simulink model "Electrical_System_2018b_obfs"  (R2019b)
settings: Solver=VariableStepAuto  StartTime=0.0  StopTime=5  RelTol=1e-3  AbsTol=1e-3  EnableMultiTasking=on
InitFcn:
  | Steady_State_Initialisation;
StopFcn:
  | %sscexplore(simlog);
  | %Logging
undefined symbols (not defined in the file): abrlhklxvp, aexgmhuedq, afmfmjnutg, afpphrjpnc, ahuxbyvruc, alarvljztt, amxnyqmnuw, aodrlwvqie, aolhmuplyq, aqpmguuqkg, auesgwirzl, aurophlnng, awamelrhru, ayfhvxflxn, azxkacuhqc, babszerikg, bawhdqanwq, bevoqecvei, bltjvqbchx, bmqsuewujl, bsmyqjfgnf, btvjbsmnve, bywgxqeadw, bziaduxaer, bzmcmdqocb, bzsvyvetat, ccsjnrbsih, cdvenygxwh, cedkrnslhx, cjheorclzs, cjrdshrtqx, ckhavyhcza, ckxewznhlz, cmrcgyiplk, conenicnws, cqkejbgjnn, csfnuwymhe, cunupkhwbh, cwzfvzuxxh, dcadmadufn, dcfponivnv, ddtrqjrhjn, dfhoxvkqas, dfrhtcwpne, dfvomcagjv, djijwylxea, dnmeqksrrm, dnzewbdkaa, dsqcykyxav, dtswwlttmm, ecumpidjtv, edegaywrct, ejjjsmnejc, eknqnehjdz, emvdetzouf, esxbqkbahr, etnkkbreiq, eunoiiiirw, ewewcuedir, fatkfxdhtc ... (+386)
libraries: fl_lib x802, ee_lib x362, fl_ps_legacy_lib x160, nesl_utility x85
(part 23 of 26)

== system Electrical_System_2018b_obfs/Redacted_1221/Redacted_7996/Redacted_9242/Redacted_38/Redacted_8107/Redacted_6003 ==
  Redacted_1930 : ee_lib/Passive/Thermal/Thermal Resistor  R=hnrivnapaq K/W  T_specify=off  T_priority=None  T=fdmzqhuwsh K  T_nominal_specify=off  T_nominal_unit=K  T_nominal_value=tdgakkaysy  Q_specify=off  Q_priority=None  Q=cbfpwknynd W  Q_nominal_specify=off  Q_nominal_unit=W  Q_nominal_value=hqcrpimszr
      settings: SourceProductName=Simscape Electrical  SourceProductBaseCode=PS  InternalSimscapePortConfiguration="{\"Bottom\":[],\"Left\":[{\"id\":\"A\",\"label\":\"A\",\"type\":\"foundation.thermal.thermal\"}],\"Right\":[{\"id\":\"B\",\"label\":\"B\",\"type\":\"foundation.thermal.thermal\"}],\"Top\":[]}"
  Redacted_2034 : ee_lib/Semiconductors & Converters/Diode  ModelType=qljxbksejb  Vf=iqtxyhzmad V  Ron=mjyptxjlpj Ohm  Goff=eaiuifgbtc S  prmExp=uovsjyapqx  I12=dfdowkcjum A  V12=mowyumyzjz V  IS=paoryjpoxj A  ec=cwojkwmiiz  I1=oyldfbivbv A  V1=dvertrfmvh V  RS=oebupxhqwy Ohm  Tmeas=latpbskjvi degC  N_series=jdrtgiwiug  N_parallel=kjrtfcnnzv  Rz=ecpdxtdyqu Ohm  BV=regbijmtbt V  C_param=crvhucdqdf  CJ=qdbprudfuu pF  CJ0=zczssgvpsu pF  VJ=fxytmivhee V  Mgrad=hqduwwifxd  Vvec=oeuqtgaaxn V  Cvec=gpqahbkocz pF  FC=siouyjskbk  Q_param=mdplkdbvxr  iRM=iffbbljxua A  iF=pfyoxsblfu A  didt=amrzuaxosg A/us  trr_factor=mnaixlwtuy  trr=zhpnzyhtrk ns  Qrr=zinteenzdg s*uA  TT=leubpgkgse ns  tau=mvtjoetwfm ns  T_param=beccsadefd  IS_T2=gikgczwyer A  I1_T2=ejowqnzasa A  V1_T2=boqexodrvc V  Tmeas2=sekozcasvt degC  EG_param=zvetvjcbns  EG=yfbumhzpta eV  XTI_param=kndiutgvbc  XTI=dmkgiicoqh  dBVdT=sjrqiebaep V/K  Tdevice=zbzjxdappo degC  i_specify=off  i_priority=None  i=pkgkjaaiux A  i_nominal_specify=off  i_nominal_unit=A  i_nominal_value=iqyazggtza  v_specify=off  v_priority=None  v=aqbrsijarw V  v_nominal_specify=off  v_nominal_unit=V  v_nominal_value=rbvnzvqoqw  i_capacitor_specify=off  i_capacitor_priority=None  i_capacitor=tuynidlyyy A  i_capacitor_nominal_specify=off  i_capacitor_nominal_unit=A  i_capacitor_nominal_value=vgeutllmom  v_capacitor_specify=off  v_capacitor_priority=None  v_capacitor=aumsjdybje V  v_capacitor_nominal_specify=off  v_capacitor_nominal_unit=V  v_capacitor_nominal_value=ylnkaqxxjx  power_dissipated_specify=off  power_dissipated_priority=None  power_dissipated=bkghkxdvlu W  power_dissipated_nominal_specify=off  power_dissipated_nominal_unit=W  power_dissipated_nominal_value=zgsnnsunjp  thermal_network_parameterization=nlxrhefnye  Rth=wenpkeadfs K/W  Rth_Foster=pmnajvgqrg K/W  thermal_mass_parameterization=bvpebdmwnx  thermal_mass=tsjtvgxgqo J/K  thermal_mass_Foster=juyxynizkb J/K  thermal_time_constant=tldqxfdatu s  thermal_time_constant_Foster=jovrtdhtnc s  thermal_mass_initial_temperatures=ikqngtdwsm degC
      settings: SourceProductName=Simscape Electrical  InternalSimscapePortConfiguration="{\"Bottom\":[],\"Left\":[{\"id\":\"p\",\"label\":\"\",\"type\":\"foundation.electrical.electrical\"},{\"id\":\"H\",\"label\":\"H\",\"type\":\"foundation.thermal.thermal\"}],\"Right\":[{\"id\":\"n\",\"label\":\"\",\"type\":\"foundation.electrical.electrical\"}],\"Top\":[]}"
  Redacted_2189 : fl_lib/Electrical/Electrical Elements/Switch  R_closed=foccbyagpm Ohm  G_open=qmhdlwyqas 1/Ohm  Threshold=mzryhutpxu  i_specify=off  i_priority=None  i=ronjclvfae A  i_nominal_specify=off  i_nominal_unit=A  i_nominal_value=pepihfswvq  v_specify=off  v_priority=None  v=riglalheal V  v_nominal_specify=off  v_nominal_unit=V  v_nominal_value=llodcbplhq
      settings: SourceProductName=Simscape
  Redacted_2683 : ee_lib/Semiconductors & Converters/Diode  ModelType=unqcuhngcz  Vf=ptgyrbybxg V  Ron=tponyfjprp Ohm  Goff=glxtjcdqxv S  prmExp=cjjxbqorob  I12=tmuirimiso A  V12=ajfpvmmvif V  IS=npqaesggkw A  ec=xhdbjedinc  I1=bhqghsexhn A  V1=kekbinqgmi V  RS=vctdzuibfy Ohm  Tmeas=ywtwqwngjn degC  N_series=ugxhiounyu  N_parallel=txdvgcjciy  Rz=prvnlkeyws Ohm  BV=wsyzieqjme V  C_param=dtqzgbyoxb  CJ=bhponiftbz pF  CJ0=lvxihytxjc pF  VJ=kcfldgdrdj V  Mgrad=ogjcpcefgy  Vvec=sngqltjsza V  Cvec=dibfbaeuxm pF  FC=qlgqcocgqi  Q_param=yhsbhadtka  iRM=vjjdgkalgm A  iF=shtzyfzyvn A  didt=hzdjajnwwy A/us  trr_factor=kikgszlwgz  trr=qxsglffrkr ns  Qrr=dtdzjmwoid s*uA  TT=hvrjrtimqi ns  tau=wsjufvhwdd ns  T_param=ieyyqxgorr  IS_T2=mxbsaftenk A  I1_T2=tkyvlqhfkw A  V1_T2=jubvikjjyh V  Tmeas2=kgfbpqicfn degC  EG_param=gliqfynxcq  EG=jzcujindyz eV  XTI_param=xhknqrejda  XTI=jxihwgswbm  dBVdT=ubhxpvgdyz V/K  Tdevice=hhsxnkxagz degC  i_specify=off  i_priority=None  i=igpuapigbx A  i_nominal_specify=off  i_nominal_unit=A  i_nominal_value=nodxoezgzy  v_specify=off  v_priority=None  v=nkzepssinp V  v_nominal_specify=off  v_nominal_unit=V  v_nominal_value=zdhnmmkhdr  i_capacitor_specify=off  i_capacitor_priority=None  i_capacitor=jiuqpxnscm A  i_capacitor_nominal_specify=off  i_capacitor_nominal_unit=A  i_capacitor_nominal_value=fsbzkpldhi  v_capacitor_specify=off  v_capacitor_priority=None  v_capacitor=wrspuopelq V  v_capacitor_nominal_specify=off  v_capacitor_nominal_unit=V  v_capacitor_nominal_value=wizxjlevyq  power_dissipated_specify=off  power_dissipated_priority=None  power_dissipated=moohbwshzg W  power_dissipated_nominal_specify=off  power_dissipated_nominal_unit=W  power_dissipated_nominal_value=orjgoavjlp  thermal_network_parameterization=vpzbbzxpak  Rth=pqattronql K/W  Rth_Foster=xvgcrkjmlg K/W  thermal_mass_parameterization=jjcteiernu  thermal_mass=nxbznqnvge J/K  thermal_mass_Foster=ykxufvckjj J/K  thermal_time_constant=jhthmobbgu s  thermal_time_constant_Foster=fxwuqslxsp s  thermal_mass_initial_temperatures=ciwlrmaqcf degC
      settings: SourceProductName=Simscape Electrical  InternalSimscapePortConfiguration="{\"Bottom\":[],\"Left\":[{\"id\":\"p\",\"label\":\"\",\"type\":\"foundation.electrical.electrical\"},{\"id\":\"H\",\"label\":\"H\",\"type\":\"foundation.thermal.thermal\"}],\"Right\":[{\"id\":\"n\",\"label\":\"\",\"type\":\"foundation.electrical.electrical\"}],\"Top\":[]}"
  Redacted_3015 : ee_lib/Passive/Thermal/Thermal Resistor  R=bsmyqjfgnf K/W  T_specify=off  T_priority=None  T=oqpnlzayxz K  T_nominal_specify=off  T_nominal_unit=K  T_nominal_value=iwtobpvuwc  Q_specify=off  Q_priority=None  Q=ktnxgmfrmp W  Q_nominal_specify=off  Q_nominal_unit=W  Q_nominal_value=upzdrzoogn
      settings: SourceProductName=Simscape Electrical  SourceProductBaseCode=PS  InternalSimscapePortConfiguration="{\"Bottom\":[],\"Left\":[{\"id\":\"A\",\"label\":\"A\",\"type\":\"foundation.thermal.thermal\"}],\"Right\":[{\"id\":\"B\",\"label\":\"B\",\"type\":\"foundation.thermal.thermal\"}],\"Top\":[]}"
  Redacted_3979 : ee_lib/Passive/Thermal/Thermal Resistor  R=rvpgyzkerd K/W  T_specify=off  T_priority=None  T=gamyhprnkw K  T_nominal_specify=off  T_nominal_unit=K  T_nominal_value=xdfqlvauja  Q_specify=off  Q_priority=None  Q=pitpazxbtg W  Q_nominal_specify=off  Q_nominal_unit=W  Q_nominal_value=xyddpdwmaj
      settings: SourceProductName=Simscape Electrical  SourceProductBaseCode=PS  InternalSimscapePortConfiguration="{\"Bottom\":[],\"Left\":[{\"id\":\"A\",\"label\":\"A\",\"type\":\"foundation.thermal.thermal\"}],\"Right\":[{\"id\":\"B\",\"label\":\"B\",\"type\":\"foundation.thermal.thermal\"}],\"Top\":[]}"
  Redacted_5139 : ee_lib/Passive/Thermal/Thermal Resistor  R=kgzasefujm K/W  T_specify=off  T_priority=None  T=glpeopccez K  T_nominal_specify=off  T_nominal_unit=K  T_nominal_value=jyjirvlwob  Q_specify=off  Q_priority=None  Q=zftpgcvoga W  Q_nominal_specify=off  Q_nominal_unit=W  Q_nominal_value=zlepoxtjjd
      settings: SourceProductName=Simscape Electrical  SourceProductBaseCode=PS  InternalSimscapePortConfiguration="{\"Bottom\":[],\"Left\":[{\"id\":\"A\",\"label\":\"A\",\"type\":\"foundation.thermal.thermal\"}],\"Right\":[{\"id\":\"B\",\"label\":\"B\",\"type\":\"foundation.thermal.thermal\"}],\"Top\":[]}"
  Redacted_5625 : fl_lib/Electrical/Electrical Elements/Switch  R_closed=hyxbklyhaw Ohm  G_open=ewgpjrxxtl 1/Ohm  Threshold=kbwhlogzhf  i_specify=off  i_priority=None  i=qjupciitbk A  i_nominal_specify=off  i_nominal_unit=A  i_nominal_value=zfpqhtzgkw  v_specify=off  v_priority=None  v=hqlzplneaj V  v_nominal_specify=off  v_nominal_unit=V  v_nominal_value=obbwqmtbii
      settings: SourceProductName=Simscape
  Redacted_5657 : ee_lib/Semiconductors & Converters/Diode  ModelType=bbawzmmnac  Vf=cfeosnswqd V  Ron=xmclnzzcel Ohm  Goff=mrxxabbkuw S  prmExp=mirycngfdn  I12=rqbalgkwyr A  V12=tabgwshiiq V  IS=ngrjfbjvvt A  ec=clnbffkkko  I1=rfqzpiiomz A  V1=xfqgijkqbu V  RS=zkaypxwvif Ohm  Tmeas=itkruelsvv degC  N_series=uufuremtuo  N_parallel=exbmquirgy  Rz=hgacsasgax Ohm  BV=bjsuhtbcxp V  C_param=auhmigqxzs  CJ=cyxjnvuiff pF  CJ0=nbcujpgwhf pF  VJ=zjdaaxugeg V  Mgrad=afzrqsjezb  Vvec=dsmzskpzrd V  Cvec=bliaftztkk pF  FC=esociklonl  Q_param=skjwelkzxv  iRM=tmfsjklyvt A  iF=cpuezbuqmz A  didt=himvddlotl A/us  trr_factor=pxnmftscld  trr=etvqnrzcrj ns  Qrr=wjswiowekh s*uA  TT=ataufdbeyn ns  tau=zrchcgagyg ns  T_param=gchzwopuhg  IS_T2=xckwpzlhlc A  I1_T2=avbcowntxa A  V1_T2=gdqqwmkozg V  Tmeas2=quzccqydmr degC  EG_param=myyrsafqxx  EG=bylhplcusy eV  XTI_param=tgzqrnxeqr  XTI=fgzgpgaqen  dBVdT=ipxpuexfni V/K  Tdevice=vftflwilyl degC  i_specify=off  i_priority=None  i=mawfnjxacl A  i_nominal_specify=off  i_nominal_unit=A  i_nominal_value=piuvggfdrd  v_specify=off  v_priority=None  v=hcyikizcwq V  v_nominal_specify=off  v_nominal_unit=V  v_nominal_value=gijzssrjyy  i_capacitor_specify=off  i_capacitor_priority=None  i_capacitor=pydmjkdgai A  i_capacitor_nominal_specify=off  i_capacitor_nominal_unit=A  i_capacitor_nominal_value=gaywohzkxq  v_capacitor_specify=off  v_capacitor_priority=None  v_capacitor=jfxdvraffy V  v_capacitor_nominal_specify=off  v_capacitor_nominal_unit=V  v_capacitor_nominal_value=vhdgjoecmz  power_dissipated_specify=off  power_dissipated_priority=None  power_dissipated=ygmcgoonkr W  power_dissipated_nominal_specify=off  power_dissipated_nominal_unit=W  power_dissipated_nominal_value=lsosbnwnhl  thermal_network_parameterization=uqxbruktsl  Rth=xaazvoxkzm K/W  Rth_Foster=ypbknnzits K/W  thermal_mass_parameterization=krtbkpmofw  thermal_mass=kqhtsapotn J/K  thermal_mass_Foster=snricxyamm J/K  thermal_time_constant=dsoiduioti s  thermal_time_constant_Foster=hjownphtlb s  thermal_mass_initial_temperatures=cbnczxkoai degC
      settings: SourceProductName=Simscape Electrical  InternalSimscapePortConfiguration="{\"Bottom\":[],\"Left\":[{\"id\":\"p\",\"label\":\"\",\"type\":\"foundation.electrical.electrical\"},{\"id\":\"H\",\"label\":\"H\",\"type\":\"foundation.thermal.thermal\"}],\"Right\":[{\"id\":\"n\",\"label\":\"\",\"type\":\"foundation.electrical.electrical\"}],\"Top\":[]}"
  Redacted_618 : ee_lib/Semiconductors & Converters/Diode  ModelType=rkpcosdcop  Vf=lzenazmxwk V  Ron=laoauccyph Ohm  Goff=eogfajxjvg S  prmExp=auhrcuewvk  I12=ephdqsweto A  V12=ybwxgsrgvn V  IS=ehwksjpkam A  ec=giupratzer  I1=shazrtegll A  V1=demzikmedl V  RS=tvlssdjwwv Ohm  Tmeas=ubohgymfpi degC  N_series=ipthgzwmna  N_parallel=bktxcarwhu  Rz=yhyrdpsjtm Ohm  BV=hfwqlzcjfg V  C_param=hapevfajvk  CJ=xwrwppuobh pF  CJ0=yyhmqjagfv pF  VJ=zdzkwausfz V  Mgrad=qxmsnreivi  Vvec=lfikgaftwv V  Cvec=xuowrvsncr pF  FC=unjvmmuvtr  Q_param=rddstsxnsr  iRM=fdsnqcchmj A  iF=fmpnloxlqx A  didt=kwjfevuvbi A/us  trr_factor=zfgybtwped  trr=xqkhnstkiy ns  Qrr=hybyujvqwm s*uA  TT=rgwrqignxd ns  tau=yyhbogviix ns  T_param=kercwremhv  IS_T2=boophnoohc A  I1_T2=acskstwime A  V1_T2=wnwbyhilui V  Tmeas2=tblacebvdl degC  EG_param=fgmqmmniev  EG=jvgkdvfiqn eV  XTI_param=tozzwxdtkj  XTI=fufkmkxntk  dBVdT=jhryqncwej V/K  Tdevice=vcluzljkyb degC  i_specify=off  i_priority=None  i=vattghsfci A  i_nominal_specify=off  i_nominal_unit=A  i_nominal_value=qbkpgcrxyx  v_specify=off  v_priority=None  v=nhxoerlgyg V  v_nominal_specify=off  v_nominal_unit=V  v_nominal_value=uyxtmtfxck  i_capacitor_specify=off  i_capacitor_priority=None  i_capacitor=yvkpdlpfsk A  i_capacitor_nominal_specify=off  i_capacitor_nominal_unit=A  i_capacitor_nominal_value=vbrriwgque  v_capacitor_specify=off  v_capacitor_priority=None  v_capacitor=rzfflaghjc V  v_capacitor_nominal_specify=off  v_capacitor_nominal_unit=V  v_capacitor_nominal_value=uwtguigmwf  power_dissipated_specify=off  power_dissipated_priority=None  power_dissipated=jrdwwynqio W  power_dissipated_nominal_specify=off  power_dissipated_nominal_unit=W  power_dissipated_nominal_value=wbkqdktlnr  thermal_network_parameterization=jpsdwhgqsa  Rth=brlvhyneff K/W  Rth_Foster=vfuijyzesi K/W  thermal_mass_parameterization=phbeyounnd  thermal_mass=dtprcnswbr J/K  thermal_mass_Foster=medownhbcv J/K  thermal_time_constant=zqahowncoh s  thermal_time_constant_Foster=wjifmgurkv s  thermal_mass_initial_temperatures=wlgtjerxmc degC
      settings: SourceProductName=Simscape Electrical  InternalSimscapePortConfiguration="{\"Bottom\":[],\"Left\":[{\"id\":\"p\",\"label\":\"\",\"type\":\"foundation.electrical.electrical\"},{\"id\":\"H\",\"label\":\"H\",\"type\":\"foundation.thermal.thermal\"}],\"Right\":[{\"id\":\"n\",\"label\":\"\",\"type\":\"foundation.electrical.electrical\"}],\"Top\":[]}"
  Redacted_713 : ee_lib/Semiconductors & Converters/Diode  ModelType=lkkcmgpbdm  Vf=bawajenmku V  Ron=kxerbojczb Ohm  Goff=omaqvwbgjm S  prmExp=mhvrvxvkqj  I12=vvcjszndgf A  V12=gwdnghxxjm V  IS=lwabrrpbjq A  ec=sqrpdlrsmb  I1=lmbkodwwso A  V1=xbfckrfhqq V  RS=expttalfyo Ohm  Tmeas=jijdjutikz degC  N_series=shguxfrayi  N_parallel=bjkplhfybw  Rz=iubaophvns Ohm  BV=yekwptqxqa V  C_param=rpswauztdx  CJ=farklfmilj pF  CJ0=sqgevuhphp pF  VJ=dlwsmbukmv V  Mgrad=dkyayzzgyw  Vvec=tsbwaimylc V  Cvec=mmqbanhdym pF  FC=tjmqolgjus  Q_param=tlwfgmybcc  iRM=dsozwffbqo A  iF=qoboxqhvid A  didt=xsxvbubgdx A/us  trr_factor=hpdsygyelk  trr=nuzrdvgkrj ns  Qrr=bidvofxoqv s*uA  TT=jbqeqqkgiu ns  tau=cdcbpkkbne ns  T_param=dqwwjegyew  IS_T2=nufxlxaznm A  I1_T2=tystfaaiyc A  V1_T2=zneeizlvme V  Tmeas2=qcubydlkcn degC  EG_param=kzeqebsucu  EG=nmfdxrvqqk eV  XTI_param=rdqutjekkf  XTI=yxstlhwzsc  dBVdT=dfsxohafhi V/K  Tdevice=tjtorimxyl degC  i_specify=off  i_priority=None  i=fyyxyedswg A  i_nominal_specify=off  i_nominal_unit=A  i_nominal_value=lvqvmsrgcq  v_specify=off  v_priority=None  v=lfxrhfhldc V  v_nominal_specify=off  v_nominal_unit=V  v_nominal_value=ahxasjhyix  i_capacitor_specify=off  i_capacitor_priority=None  i_capacitor=sxezhempdb A  i_capacitor_nominal_specify=off  i_capacitor_nominal_unit=A  i_capacitor_nominal_value=oleoyenlww  v_capacitor_specify=off  v_capacitor_priority=None  v_capacitor=vkfdkqfqeh V  v_capacitor_nominal_specify=off  v_capacitor_nominal_unit=V  v_capacitor_nominal_value=sppyhpvyds  power_dissipated_specify=off  power_dissipated_priority=None  power_dissipated=qxpynkfasn W  power_dissipated_nominal_specify=off  power_dissipated_nominal_unit=W  power_dissipated_nominal_value=wuwbigxvpe  thermal_network_parameterization=vnxrsoiwal  Rth=xnfauzfygo K/W  Rth_Foster=omfzlihdit K/W  thermal_mass_parameterization=vyjchpsxmq  thermal_mass=jkxmnrnghg J/K  thermal_mass_Foster=voiyfowxdv J/K  thermal_time_constant=sluohzzprg s  thermal_time_constant_Foster=hfrqbgktbf s  thermal_mass_initial_temperatures=oxayzqemir degC
      settings: SourceProductName=Simscape Electrical  InternalSimscapePortConfiguration="{\"Bottom\":[],\"Left\":[{\"id\":\"p\",\"label\":\"\",\"type\":\"foundation.electrical.electrical\"},{\"id\":\"H\",\"label\":\"H\",\"type\":\"foundation.thermal.thermal\"}],\"Right\":[{\"id\":\"n\",\"label\":\"\",\"type\":\"foundation.electrical.electrical\"}],\"Top\":[]}"
  Redacted_8101 : ee_lib/Semiconductors & Converters/Diode  ModelType=vjvfilmehi  Vf=uqqnuzepqx V  Ron=avqhenjvsv Ohm  Goff=rtumjurihv S  prmExp=uigzpzscli  I12=vzjzhllkvk A  V12=ojjywpkmgq V  IS=ncftzddrsj A  ec=gqxfqbvlbn  I1=hnezitzofg A  V1=xyfwatnudk V  RS=qcfzyruown Ohm  Tmeas=vfdobhlqgn degC  N_series=vqbwovlfee  N_parallel=zgbdyhlnre  Rz=excquvkvhq Ohm  BV=ytokprdnyg V  C_param=ucbqghdhxa  CJ=dvwvqhnfff pF  CJ0=frpzzolkvk pF  VJ=pawvicfbbc V  Mgrad=ypwhnnyrsu  Vvec=uicrbrruuj V  Cvec=wtiolrfbff pF  FC=aunplnfgfp  Q_param=gvkigwoccs  iRM=wvnjtfcgby A  iF=nqysjagfvv A  didt=rkunyesksy A/us  trr_factor=lwitxjrpgi  trr=puwjytdnut ns  Qrr=dqzfqmjjjs s*uA  TT=stjztyrfdv ns  tau=wfpwkdmppl ns  T_param=jcnwbtzkcv  IS_T2=lprsqxbaio A  I1_T2=srzmfqmede A  V1_T2=jqjcmaaijo V  Tmeas2=njdkhnpwzi degC  EG_param=dfjweqxukn  EG=ruwbtenrdr eV  XTI_param=qsgfuzyxoi  XTI=pzhtmlrafz  dBVdT=lahtjyboks V/K  Tdevice=qjeiploltt degC  i_specify=off  i_priority=None  i=ozlejdjjmp A  i_nominal_specify=off  i_nominal_unit=A  i_nominal_value=qdymktiybr  v_specify=off  v_priority=None  v=vnzfcfcuel V  v_nominal_specify=off  v_nominal_unit=V  v_nominal_value=hjcwyunqcl  i_capacitor_specify=off  i_capacitor_priority=None  i_capacitor=pgogaxptoz A  i_capacitor_nominal_specify=off  i_capacitor_nominal_unit=A  i_capacitor_nominal_value=oxnlvytclw  v_capacitor_specify=off  v_capacitor_priority=None  v_capacitor=muyrsrrbwr V  v_capacitor_nominal_specify=off  v_capacitor_nominal_unit=V  v_capacitor_nominal_value=zlvcwbvrnn  power_dissipated_specify=off  power_dissipated_priority=None  power_dissipated=ghecyltvbi W  power_dissipated_nominal_specify=off  power_dissipated_nominal_unit=W  power_dissipated_nominal_value=wlpqqofirg  thermal_network_parameterization=tglpwybeup  Rth=ryhjudbnet K/W  Rth_Foster=lkfeyvluqb K/W  thermal_mass_parameterization=xurnjbxmdo  thermal_mass=dprmjamjnx J/K  thermal_mass_Foster=uvzmwxcsfs J/K  thermal_time_constant=tltzvjscxf s  thermal_time_constant_Foster=kwxfnvsffq s  thermal_mass_initial_temperatures=njohwjfpww degC
      settings: SourceProductName=Simscape Electrical  InternalSimscapePortConfiguration="{\"Bottom\":[],\"Left\":[{\"id\":\"p\",\"label\":\"\",\"type\":\"foundation.electrical.electrical\"},{\"id\":\"H\",\"label\":\"H\",\"type\":\"foundation.thermal.thermal\"}],\"Right\":[{\"id\":\"n\",\"label\":\"\",\"type\":\"foundation.electrical.electrical\"}],\"Top\":[]}"
  Redacted_8530 : fl_lib/Electrical/Electrical Elements/Switch  R_closed=rejrngwejd Ohm  G_open=yiexqkczmq 1/Ohm  Threshold=recrphtyvw  i_specify=off  i_priority=None  i=buwhhqhusz A  i_nominal_specify=off  i_nominal_unit=A  i_nominal_value=okhgulhtsx  v_specify=off  v_priority=None  v=cplpfmpzdf V  v_nominal_specify=off  v_nominal_unit=V  v_nominal_value=jgoyagttqd
      settings: SourceProductName=Simscape
  Redacted_3998 : PMIOPort  Side=Left
  Redacted_2949 : PMIOPort  Port=2  Side=Left
  Redacted_7751 : PMIOPort  Port=3  Side=Left
  Redacted_2080 : PMIOPort  Port=4  Side=Right
  Redacted_919 : PMIOPort  Port=5  Side=Right
  Redacted_5475 : PMIOPort  Port=6  Side=Right
  Redacted_7661 : PMIOPort  Port=7  Side=Left
  Redacted_3448 : PMIOPort  Port=8  Side=Right
  connections:
  Redacted_8101/LConn1 -- Redacted_2949/RConn1 -- Redacted_618/RConn1
  Redacted_8101/RConn1 -- Redacted_5625/LConn1 -- Redacted_618/LConn1
  Redacted_5139/LConn1 -- Redacted_5657/LConn2 -- Redacted_2034/LConn2
  Redacted_2080/RConn1 -- Redacted_8530/RConn2
  Redacted_2034/LConn1 -- Redacted_8530/LConn1 -- Redacted_5657/RConn1
  Redacted_5657/LConn1 -- Redacted_3998/RConn1 -- Redacted_2034/RConn1
  Redacted_1930/RConn1 -- Redacted_3979/RConn1 -- Redacted_3015/LConn1 -- Redacted_5139/RConn1
  Redacted_2683/LConn1 -- Redacted_7751/RConn1 -- Redacted_713/RConn1
  Redacted_5475/RConn1 -- Redacted_2189/RConn2
  Redacted_3448/RConn1 -- Redacted_2189/RConn1 -- Redacted_5625/RConn1 -- Redacted_8530/RConn1
  Redacted_919/RConn1 -- Redacted_5625/RConn2
  Redacted_713/LConn1 -- Redacted_2189/LConn1 -- Redacted_2683/RConn1
  Redacted_713/LConn2 -- Redacted_3979/LConn1 -- Redacted_2683/LConn2
  Redacted_3015/RConn1 -- Redacted_7661/RConn1
  Redacted_8101/LConn2 -- Redacted_618/LConn2 -- Redacted_1930/LConn1

== system Electrical_System_2018b_obfs/Redacted_1221/Redacted_7996/Redacted_9242/Redacted_38/Redacted_8107/Redacted_6242 ==
  Redacted_2327 : ee_lib/Semiconductors & Converters/Diode  ModelType=zlqozpkodf  Vf=xnmadrvlcd V  Ron=uunrbpulhg Ohm  Goff=xsfjcpkxqq S  prmExp=ilzhmxhuaq  I12=gyasufgvuq A  V12=idjookybuc V  IS=bcffcwsapx A  ec=pihedtkusy  I1=kwzjqxggxg A  V1=pbzkicbjfn V  RS=wdatpkrqkc Ohm  Tmeas=hvyhqfvdcb degC  N_series=alyiitrfrm  N_parallel=slhahnjxxj  Rz=ruhhhlvmhe Ohm  BV=ufrdribnqb V  C_param=ublgvuqudh  CJ=wjimkqwodx pF  CJ0=wbyejgyhoo pF  VJ=rjkklxlhsj V  Mgrad=phvcsjstwm  Vvec=ueprrqizyd V  Cvec=veksrfdunv pF  FC=kteqfykfjf  Q_param=lwtzvkdmhq  iRM=edafgvdbbh A  iF=webvhcrhgo A  didt=dyksqyphqg A/us  trr_factor=lsneluuczu  trr=qxgopfrsuu ns  Qrr=dppwwseqii s*uA  TT=fvnsmamjqw ns  tau=coqdaramvm ns  T_param=vnptnkvrrw  IS_T2=ktfizonbgf A  I1_T2=ghckxllgao A  V1_T2=geuiycovwc V  Tmeas2=tjlqxwblyr degC  EG_param=milzlladvp  EG=pedjbioglz eV  XTI_param=qovocfshmo  XTI=prcytdsldj  dBVdT=sowvegegbn V/K  Tdevice=byhsjhmdht degC  i_specify=off  i_priority=None  i=zhhbbcahbl A  i_nominal_specify=off  i_nominal_unit=A  i_nominal_value=oryudlxkyl  v_specify=off  v_priority=None  v=odphdlkqwc V  v_nominal_specify=off  v_nominal_unit=V  v_nominal_value=uwyzcweltx  i_capacitor_specify=off  i_capacitor_priority=None  i_capacitor=dmacsdhbbs A  i_capacitor_nominal_specify=off  i_capacitor_nominal_unit=A  i_capacitor_nominal_value=ybcyxnellk  v_capacitor_specify=off  v_capacitor_priority=None  v_capacitor=vpnohamqui V  v_capacitor_nominal_specify=off  v_capacitor_nominal_unit=V  v_capacitor_nominal_value=gjkqvvfuhx  power_dissipated_specify=off  power_dissipated_priority=None  power_dissipated=isecubhovm W  power_dissipated_nominal_specify=off  power_dissipated_nominal_unit=W  power_dissipated_nominal_value=xvxirfhpyu  thermal_network_parameterization=bgokhfhnzu  Rth=xpxrmgvwvl K/W  Rth_Foster=oufrqiugec K/W  thermal_mass_parameterization=zxpnysspsw  thermal_mass=zwmkkpurfv J/K  thermal_mass_Foster=btycqmhagw J/K  thermal_time_constant=ewaeisnjee s  thermal_time_constant_Foster=tzmkbuadoh s  thermal_mass_initial_temperatures=ltruoavqyb degC
      settings: SourceProductName=Simscape Electrical  InternalSimscapePortConfiguration="{\"Bottom\":[],\"Left\":[{\"id\":\"p\",\"label\":\"\",\"type\":\"foundation.electrical.electrical\"},{\"id\":\"H\",\"label\":\"H\",\"type\":\"foundation.thermal.thermal\"}],\"Right\":[{\"id\":\"n\",\"label\":\"\",\"type\":\"foundation.electrical.electrical\"}],\"Top\":[]}"
  Redacted_2962 : ee_lib/Semiconductors & Converters/Diode  ModelType=jjrheygjsy  Vf=vlxfhtkcow V  Ron=evsurbtjfl Ohm  Goff=qevbfhcokp S  prmExp=dnrbutsija  I12=bnmtmmbcgm A  V12=shyycjhzns V  IS=azxolkbjym A  ec=tezwxmnvpl  I1=sifcyqltlj A  V1=pqnfmmqkjs V  RS=fvxpukthko Ohm  Tmeas=mudxvsbldr degC  N_series=raoxyfqegz  N_parallel=voupkjcdms  Rz=cmksowdtvm Ohm  BV=risztpwwnb V  C_param=nrfnpggenx  CJ=uowzsywqxj pF  CJ0=sojkfcdtip pF  VJ=gabqrztkww V  Mgrad=jzlxzlqafl  Vvec=vzciixfpkg V  Cvec=bsgfoapyas pF  FC=tarcipquxd  Q_param=edmkxpfaxm  iRM=qutcvtcfxw A  iF=vmbyklghxw A  didt=pucxkdozsm A/us  trr_factor=wzmyanqqyk  trr=tdyyhqwywf ns  Qrr=ketbbqwbvn s*uA  TT=ghehbiqbqm ns  tau=wrowrqpdff ns  T_param=gsyyvoqdlk  IS_T2=mnkjvixzgv A  I1_T2=fmopzwtayx A  V1_T2=rfpmzpboqu V  Tmeas2=hoyeidagap degC  EG_param=mdpweemffq  EG=gwrcmykbqb eV  XTI_param=drvljlyowh  XTI=tzgjofrmtk  dBVdT=erfpmvnhnt V/K  Tdevice=auexbqhlak degC  i_specify=off  i_priority=None  i=vhaglczhfm A  i_nominal_specify=off  i_nominal_unit=A  i_nominal_value=wfbbfbsxrj  v_specify=off  v_priority=None  v=xntcrpsqrk V  v_nominal_specify=off  v_nominal_unit=V  v_nominal_value=fdcfxeezjy  i_capacitor_specify=off  i_capacitor_priority=None  i_capacitor=qhxvpsgxps A  i_capacitor_nominal_specify=off  i_capacitor_nominal_unit=A  i_capacitor_nominal_value=jpqlrlmgjj  v_capacitor_specify=off  v_capacitor_priority=None  v_capacitor=lspvwmjgec V  v_capacitor_nominal_specify=off  v_capacitor_nominal_unit=V  v_capacitor_nominal_value=pdcnizlbjj  power_dissipated_specify=off  power_dissipated_priority=None  power_dissipated=izflmcaxys W  power_dissipated_nominal_specify=off  power_dissipated_nominal_unit=W  power_dissipated_nominal_value=fdwizxacwl  thermal_network_parameterization=cjjbjjpkfc  Rth=fuckyjlkdp K/W  Rth_Foster=jxeypfldhg K/W  thermal_mass_parameterization=uohxvxswjw  thermal_mass=asbxvaopib J/K  thermal_mass_Foster=jttgemwnfa J/K  thermal_time_constant=zspqfjgjgz s  thermal_time_constant_Foster=ilamkzrgce s  thermal_mass_initial_temperatures=xhwrtwekqg degC
      settings: SourceProductName=Simscape Electrical  InternalSimscapePortConfiguration="{\"Bottom\":[],\"Left\":[{\"id\":\"p\",\"label\":\"\",\"type\":\"foundation.electrical.electrical\"},{\"id\":\"H\",\"label\":\"H\",\"type\":\"foundation.thermal.thermal\"}],\"Right\":[{\"id\":\"n\",\"label\":\"\",\"type\":\"foundation.electrical.electrical\"}],\"Top\":[]}"
  Redacted_3070 : ee_lib/Passive/Thermal/Thermal Resistor  R=wiqttwajce K/W  T_specify=off  T_priority=None  T=vqrtwscryb K  T_nominal_specify=off  T_nominal_unit=K  T_nominal_value=zvetejgzmy  Q_specify=off  Q_priority=None  Q=hbvniwvmxr W  Q_nominal_specify=off  Q_nominal_unit=W  Q_nominal_value=ddjhqnqmyp
      settings: SourceProductName=Simscape Electrical  SourceProductBaseCode=PS  InternalSimscapePortConfiguration="{\"Bottom\":[],\"Left\":[{\"id\":\"A\",\"label\":\"A\",\"type\":\"foundation.thermal.thermal\"}],\"Right\":[{\"id\":\"B\",\"label\":\"B\",\"type\":\"foundation.thermal.thermal\"}],\"Top\":[]}"
  Redacted_3625 : fl_lib/Electrical/Electrical Elements/Switch  R_closed=seoolmwehr Ohm  G_open=hxonowfndl 1/Ohm  Threshold=pamymdveox  i_specify=off  i_priority=None  i=zrvvhzvjff A  i_nominal_specify=off  i_nominal_unit=A  i_nominal_value=ibonwfjjgh  v_specify=off  v_priority=None  v=nnojsmmnqo V  v_nominal_specify=off  v_nominal_unit=V  v_nominal_value=lccejxhfzy
      settings: SourceProductName=Simscape
  Redacted_4987 : fl_lib/Electrical/Electrical Elements/Switch  R_closed=lhkszjvyjj Ohm  G_open=cfmhwocoqg 1/Ohm  Threshold=wrdozfjgks  i_specify=off  i_priority=None  i=vxlbhcczxq A  i_nominal_specify=off  i_nominal_unit=A  i_nominal_value=qwnospzsor  v_specify=off  v_priority=None  v=xftjvfsoez V  v_nominal_specify=off  v_nominal_unit=V  v_nominal_value=gumzwtwaow
      settings: SourceProductName=Simscape
  Redacted_5889 : ee_lib/Semiconductors & Converters/Diode  ModelType=lmninslupp  Vf=csvrgbpymj V  Ron=rwgttififz Ohm  Goff=khfoyorwul S  prmExp=syzdajwpfj  I12=cklseiaeez A  V12=swobehblec V  IS=gmanpopldp A  ec=ubainqujzq  I1=hnhtgdqgkb A  V1=tlybrivvuq V  RS=ahjwdmfbvz Ohm  Tmeas=wvcilsaecx degC  N_series=kvfdoalkva  N_parallel=rshtgefppy  Rz=upovawayzb Ohm  BV=rnlhrkanwf V  C_param=jivgjpocjh  CJ=pyzjtgvamu pF  CJ0=eqfsxlrklc pF  VJ=arahunfjhp V  Mgrad=ueczlzcnat  Vvec=veaokirrga V  Cvec=kaoibdnzse pF  FC=mzpqxmpqpr  Q_param=vceuukrpaf  iRM=menolzglxm A  iF=lmazalwvlj A  didt=mrucchcqzp A/us  trr_factor=jmqbegzwyd  trr=epdgjzyruk ns  Qrr=arnefhstmd s*uA  TT=uqcixasjsm ns  tau=deccqtnhsg ns  T_param=zohwtnmcxb  IS_T2=cqnkuqeokv A  I1_T2=swffggghol A  V1_T2=szzjwjwpqt V  Tmeas2=ozbikfpfll degC  EG_param=urvuhvgoko  EG=tnjfalvupd eV  XTI_param=pwfsfgkrme  XTI=deppuugfiu  dBVdT=drqiecenop V/K  Tdevice=rfsnkzbyux degC  i_specify=off  i_priority=None  i=biojvuxxwk A  i_nominal_specify=off  i_nominal_unit=A  i_nominal_value=dwbfbzrsfp  v_specify=off  v_priority=None  v=efdhnjbiac V  v_nominal_specify=off  v_nominal_unit=V  v_nominal_value=kigzumhtda  i_capacitor_specify=off  i_capacitor_priority=None  i_capacitor=uolwwpldjl A  i_capacitor_nominal_specify=off  i_capacitor_nominal_unit=A  i_capacitor_nominal_value=ruzowqbsei  v_capacitor_specify=off  v_capacitor_priority=None  v_capacitor=vyczpjjfws V  v_capacitor_nominal_specify=off  v_capacitor_nominal_unit=V  v_capacitor_nominal_value=bjdjcopbwt  power_dissipated_specify=off  power_dissipated_priority=None  power_dissipated=lihsuptkrc W  power_dissipated_nominal_specify=off  power_dissipated_nominal_unit=W  power_dissipated_nominal_value=kidbfkbtre  thermal_network_parameterization=jmpugmicww  Rth=sqcxlhkapl K/W  Rth_Foster=axrqtdretb K/W  thermal_mass_parameterization=kpjiseswqh  thermal_mass=hrkzeezvjd J/K  thermal_mass_Foster=gagwbgdusw J/K  thermal_time_constant=mqagdgywen s  thermal_time_constant_Foster=liitnumvzc s  thermal_mass_initial_temperatures=pktxmtgnmv degC
      settings: SourceProductName=Simscape Electrical  InternalSimscapePortConfiguration="{\"Bottom\":[],\"Left\":[{\"id\":\"p\",\"label\":\"\",\"type\":\"foundation.electrical.electrical\"},{\"id\":\"H\",\"label\":\"H\",\"type\":\"foundation.thermal.thermal\"}],\"Right\":[{\"id\":\"n\",\"label\":\"\",\"type\":\"foundation.electrical.electrical\"}],\"Top\":[]}"
  Redacted_6471 : ee_lib/Passive/Thermal/Thermal Resistor  R=stegwtgrmu K/W  T_specify=off  T_priority=None  T=jtxznumaqv K  T_nominal_specify=off  T_nominal_unit=K  T_nominal_value=xgiqpfmikh  Q_specify=off  Q_priority=None  Q=huuwcyppeg W  Q_nominal_specify=off  Q_nominal_unit=W  Q_nominal_value=ziosklkfan
      settings: SourceProductName=Simscape Electrical  SourceProductBaseCode=PS  InternalSimscapePortConfiguration="{\"Bottom\":[],\"Left\":[{\"id\":\"A\",\"label\":\"A\",\"type\":\"foundation.thermal.thermal\"}],\"Right\":[{\"id\":\"B\",\"label\":\"B\",\"type\":\"foundation.thermal.thermal\"}],\"Top\":[]}"
  Redacted_7186 : ee_lib/Semiconductors & Converters/Diode  ModelType=vzpckcvqyc  Vf=nxsxqadxmc V  Ron=ilnawabueo Ohm  Goff=stxdpoctxz S  prmExp=ununwhhxby  I12=svymktsczy A  V12=oegajdmnyb V  IS=lbbdcuffxg A  ec=udwjqsgpjf  I1=ybeycvmzsy A  V1=dqfjimonsf V  RS=mssadeassj Ohm  Tmeas=gezoccvntx degC  N_series=zfzzwnrkgr  N_parallel=jgraxkiwhn  Rz=spinfmmkte Ohm  BV=zwfovhwntt V  C_param=gvjdaupfos  CJ=zxcqjuyemq pF  CJ0=lniunuifhy pF  VJ=lcygjcqwnt V  Mgrad=anaotfathz  Vvec=vfqkviyvbe V  Cvec=tcekygpxmx pF  FC=urbxjpfufd  Q_param=yzrwoslcxv  iRM=gukblxnmqz A  iF=nlkyzmqnok A  didt=eenokvzgkp A/us  trr_factor=nngtmruros  trr=pbepfoydpp ns  Qrr=ofyeaovqye s*uA  TT=ntkcphmlia ns  tau=rasivivzfr ns  T_param=cckzsbhjwp  IS_T2=ktgtjlpbpx A  I1_T2=vvdhoydvdj A  V1_T2=myuecmejho V  Tmeas2=okrbjnkvap degC  EG_param=ceixentrzp  EG=levaozafvx eV  XTI_param=pgwlklpexk  XTI=jyhcpdepnx  dBVdT=ayyyjqgset V/K  Tdevice=mgcdqpnbuq degC  i_specify=off  i_priority=None  i=ymzagwsgrh A  i_nominal_specify=off  i_nominal_unit=A  i_nominal_value=qbyoiypxwd  v_specify=off  v_priority=None  v=lcjizkauud V  v_nominal_specify=off  v_nominal_unit=V  v_nominal_value=htzlivrmwe  i_capacitor_specify=off  i_capacitor_priority=None  i_capacitor=jmdqcbirga A  i_capacitor_nominal_specify=off  i_capacitor_nominal_unit=A  i_capacitor_nominal_value=pzfktenlhj  v_capacitor_specify=off  v_capacitor_priority=None  v_capacitor=qnligafvyc V  v_capacitor_nominal_specify=off  v_capacitor_nominal_unit=V  v_capacitor_nominal_value=gbsdjpsozv  power_dissipated_specify=off  power_dissipated_priority=None  power_dissipated=bmbnmqoutv W  power_dissipated_nominal_specify=off  power_dissipated_nominal_unit=W  power_dissipated_nominal_value=tjrgafdsiz  thermal_network_parameterization=xwefqzdezr  Rth=tfwfmrgmtu K/W  Rth_Foster=eicdrsqcji K/W  thermal_mass_parameterization=yrytmeuisg  thermal_mass=slducblorv J/K  thermal_mass_Foster=qcqbjmwgop J/K  thermal_time_constant=tgmcjvkujh s  thermal_time_constant_Foster=ouvbmdmarv s  thermal_mass_initial_temperatures=jxchskgvjo degC
      settings: SourceProductName=Simscape Electrical  InternalSimscapePortConfiguration="{\"Bottom\":[],\"Left\":[{\"id\":\"p\",\"label\":\"\",\"type\":\"foundation.electrical.electrical\"},{\"id\":\"H\",\"label\":\"H\",\"type\":\"foundation.thermal.thermal\"}],\"Right\":[{\"id\":\"n\",\"label\":\"\",\"type\":\"foundation.electrical.electrical\"}],\"Top\":[]}"
  Redacted_8807 : ee_lib/Passive/Thermal/Thermal Resistor  R=hxnldywwpo K/W  T_specify=off  T_priority=None  T=nzwtmokxjw K  T_nominal_specify=off  T_nominal_unit=K  T_nominal_value=wpvmkohsyo  Q_specify=off  Q_priority=None  Q=gcolguzwgv W  Q_nominal_specify=off  Q_nominal_unit=W  Q_nominal_value=mciyiwbijt
      settings: SourceProductName=Simscape Electrical  SourceProductBaseCode=PS  InternalSimscapePortConfiguration="{\"Bottom\":[],\"Left\":[{\"id\":\"A\",\"label\":\"A\",\"type\":\"foundation.thermal.thermal\"}],\"Right\":[{\"id\":\"B\",\"label\":\"B\",\"type\":\"foundation.thermal.thermal\"}],\"Top\":[]}"
  Redacted_8675 : PMIOPort  Side=Left
  Redacted_8577 : PMIOPort  Port=2  Side=Right
  Redacted_9694 : PMIOPort  Port=3  Side=Left
  Redacted_9591 : PMIOPort  Port=4  Side=Right
  Redacted_6570 : PMIOPort  Port=5  Side=Left
  Redacted_9250 : PMIOPort  Port=6  Side=Right
  connections:
  Redacted_7186/LConn2 -- Redacted_2962/LConn2 -- Redacted_6471/LConn1
  Redacted_8807/RConn1 -- Redacted_6570/RConn1
  Redacted_5889/LConn2 -- Redacted_2327/LConn2 -- Redacted_3070/LConn1
  Redacted_7186/RConn1 -- Redacted_8675/RConn1 -- Redacted_2962/LConn1
  Redacted_2962/RConn1 -- Redacted_4987/LConn1 -- Redacted_7186/LConn1
  Redacted_8577/RConn1 -- Redacted_4987/RConn2
  Redacted_3625/RConn1 -- Redacted_9250/RConn1 -- Redacted_4987/RConn1
  Redacted_9591/RConn1 -- Redacted_3625/RConn2
  Redacted_8807/LConn1 -- Redacted_3070/RConn1 -- Redacted_6471/RConn1
  Redacted_2327/RConn1 -- Redacted_9694/RConn1 -- Redacted_5889/LConn1
  Redacted_5889/RConn1 -- Redacted_2327/LConn1 -- Redacted_3625/LConn1

== system Electrical_System_2018b_obfs/Redacted_1221/Redacted_7996/Redacted_9242/Redacted_38/Redacted_8107/Redacted_7463 ==
  Redacted_1380 : ee_lib/Passive/Thermal/Thermal Resistor  R=bltjvqbchx K/W  T_specify=off  T_priority=None  T=vjsulqijdu K  T_nominal_specify=off  T_nominal_unit=K  T_nominal_value=ekqgnjqlcs  Q_specify=off  Q_priority=None  Q=ynempikuve W  Q_nominal_specify=off  Q_nominal_unit=W  Q_nominal_value=usndbvujjd
      settings: SourceProductName=Simscape Electrical  SourceProductBaseCode=PS  InternalSimscapePortConfiguration="{\"Bottom\":[],\"Left\":[{\"id\":\"A\",\"label\":\"A\",\"type\":\"foundation.thermal.thermal\"}],\"Right\":[{\"id\":\"B\",\"label\":\"B\",\"type\":\"foundation.thermal.thermal\"}],\"Top\":[]}"
  Redacted_1604 : ee_lib/Semiconductors & Converters/Diode  ModelType=qzjyqhdmvi  Vf=lovsephbqe V  Ron=tlypypedur Ohm  Goff=uldwabiusp S  prmExp=egkwpysxlz  I12=lwqpaixpfl A  V12=gfyywvxbpe V  IS=yxlxfqpzif A  ec=xfhtcekplz  I1=ubwdkpliwn A  V1=gdegqbtxzj V  RS=ubjqvopphy Ohm  Tmeas=xzyjlxujlg degC  N_series=uhyjtaegjn  N_parallel=dovtoubbuj  Rz=zqqzyiqjol Ohm  BV=zkuwtjkgge V  C_param=atbyjmqwkf  CJ=skadagvmew pF  CJ0=bnlwsekdxp pF  VJ=baaxjluctq V  Mgrad=icddhqsyen  Vvec=hrgnvjjanl V  Cvec=gdxzygzjqx pF  FC=cohzovhzst  Q_param=ohaajunfoi  iRM=ykhrcwmwed A  iF=woxkklqrdv A  didt=fftvjgecyz A/us  trr_factor=lletvasnhi  trr=gzuuvmcsky ns  Qrr=raghmbywvg s*uA  TT=cayllkezty ns  tau=gcxyrgecjz ns  T_param=nxmsihhosw  IS_T2=dwjvywjzly A  I1_T2=rfmrbudweq A  V1_T2=azigtcolbm V  Tmeas2=oifahqdsyj degC  EG_param=oxznrujiuq  EG=sgqrwmfyoi eV  XTI_param=enmfigzyuz  XTI=gltbrrprzn  dBVdT=zajfvnsucw V/K  Tdevice=wikizywhlb degC  i_specify=off  i_priority=None  i=lmosefjhuj A  i_nominal_specify=off  i_nominal_unit=A  i_nominal_value=nfnbjizyow  v_specify=off  v_priority=None  v=nqyjmdafen V  v_nominal_specify=off  v_nominal_unit=V  v_nominal_value=lqohnznhvt  i_capacitor_specify=off  i_capacitor_priority=None  i_capacitor=gutmqltiah A  i_capacitor_nominal_specify=off  i_capacitor_nominal_unit=A  i_capacitor_nominal_value=wyptvnsiie  v_capacitor_specify=off  v_capacitor_priority=None  v_capacitor=wrdgnruljd V  v_capacitor_nominal_specify=off  v_capacitor_nominal_unit=V  v_capacitor_nominal_value=rncavkypay  power_dissipated_specify=off  power_dissipated_priority=None  power_dissipated=fsvklglstm W  power_dissipated_nominal_specify=off  power_dissipated_nominal_unit=W  power_dissipated_nominal_value=qvokvzseij  thermal_network_parameterization=bfpwgdmmpu  Rth=lxllqemzrc K/W  Rth_Foster=aomnunguqu K/W  thermal_mass_parameterization=dmtmkrkhox  thermal_mass=juamuzkjtb J/K  thermal_mass_Foster=iferjczhav J/K  thermal_time_constant=jrxmrgjsgk s  thermal_time_constant_Foster=toaagpfobt s  thermal_mass_initial_temperatures=pdhsujzony degC
      settings: SourceProductName=Simscape Electrical  InternalSimscapePortConfiguration="{\"Bottom\":[],\"Left\":[{\"id\":\"p\",\"label\":\"\",\"type\":\"foundation.electrical.electrical\"},{\"id\":\"H\",\"label\":\"H\",\"type\":\"foundation.thermal.thermal\"}],\"Right\":[{\"id\":\"n\",\"label\":\"\",\"type\":\"foundation.electrical.electrical\"}],\"Top\":[]}"
  Redacted_2923 : ee_lib/Semiconductors & Converters/Diode  ModelType=fxjpxifjkw  Vf=noexjmbakf V  Ron=jkkshvnkns Ohm  Goff=ywhnakjquv S  prmExp=nmvmmfncnw  I12=kxageaudwl A  V12=vlioisiqjv V  IS=pedwhqxves A  ec=taciqeqolo  I1=kbxiutyaey A  V1=uneeqdstmi V  RS=sgllwkmhbl Ohm  Tmeas=bzypyozqhw degC  N_series=nrxacspjqq  N_parallel=qfmqthorqo  Rz=nodbybymfq Ohm  BV=eyuuvdyjhv V  C_param=npxkjiyocm  CJ=wpxbqjchih pF  CJ0=cbldrsoaiz pF  VJ=osklhfbdrp V  Mgrad=kqdjbouxoz  Vvec=pwwozdaaqz V  Cvec=hlkmhlwdem pF  FC=oedhbxmrxz  Q_param=khwnuzkwyi  iRM=nhbjwxxpgp A  iF=simcqbdgmi A  didt=ovzwqanxpf A/us  trr_factor=evuqdftbxj  trr=jcqvmahrea ns  Qrr=oktlohrjzb s*uA  TT=gvlcjvobly ns  tau=qetirjodwa ns  T_param=mszhnhfygj  IS_T2=pxpkyuueyv A  I1_T2=jwxglqtzpk A  V1_T2=sdzdcxyyov V  Tmeas2=qiwmtgikso degC  EG_param=yaltcbziko  EG=qakqwvlcwd eV  XTI_param=sfcevwaumy  XTI=gzyeixomgs  dBVdT=bcyojqafzz V/K  Tdevice=fisheuznsz degC  i_specify=off  i_priority=None  i=fxxjnfxjaj A  i_nominal_specify=off  i_nominal_unit=A  i_nominal_value=kroloenmzd  v_specify=off  v_priority=None  v=bxlurisorw V  v_nominal_specify=off  v_nominal_unit=V  v_nominal_value=irbwwpkiyk  i_capacitor_specify=off  i_capacitor_priority=None  i_capacitor=urgwrxpwfe A  i_capacitor_nominal_specify=off  i_capacitor_nominal_unit=A  i_capacitor_nominal_value=yybbrgcoth  v_capacitor_specify=off  v_capacitor_priority=None  v_capacitor=uptsmraffn V  v_capacitor_nominal_specify=off  v_capacitor_nominal_unit=V  v_capacitor_nominal_value=iyetwimeld  power_dissipated_specify=off  power_dissipated_priority=None  power_dissipated=queftxxrlz W  power_dissipated_nominal_specify=off  power_dissipated_nominal_unit=W  power_dissipated_nominal_value=yffwavjdoh  thermal_network_parameterization=zkwkaikjgf  Rth=cvhhawlvah K/W  Rth_Foster=szbzjrnebj K/W  thermal_mass_parameterization=kjhdyminvt  thermal_mass=xsmrpwztmg J/K  thermal_mass_Foster=mcdwbczime J/K  thermal_time_constant=wqydvlrecb s  thermal_time_constant_Foster=scwrfiazlq s  thermal_mass_initial_temperatures=lgkfgbafgg degC
      settings: SourceProductName=Simscape Electrical  InternalSimscapePortConfiguration="{\"Bottom\":[],\"Left\":[{\"id\":\"p\",\"label\":\"\",\"type\":\"foundation.electrical.electrical\"},{\"id\":\"H\",\"label\":\"H\",\"type\":\"foundation.thermal.thermal\"}],\"Right\":[{\"id\":\"n\",\"label\":\"\",\"type\":\"foundation.electrical.electrical\"}],\"Top\":[]}"
  Redacted_3309 : ee_lib/Passive/Thermal/Thermal Resistor  R=hpmnofrura K/W  T_specify=off  T_priority=None  T=sggocxblvp K  T_nominal_specify=off  T_nominal_unit=K  T_nominal_value=oihdbzxowj  Q_specify=off  Q_priority=None  Q=mdionudvgi W  Q_nominal_specify=off  Q_nominal_unit=W  Q_nominal_value=huzzujwzof
      settings: SourceProductName=Simscape Electrical  SourceProductBaseCode=PS  InternalSimscapePortConfiguration="{\"Bottom\":[],\"Left\":[{\"id\":\"A\",\"label\":\"A\",\"type\":\"foundation.thermal.thermal\"}],\"Right\":[{\"id\":\"B\",\"label\":\"B\",\"type\":\"foundation.thermal.thermal\"}],\"Top\":[]}"
  Redacted_3785 : fl_lib/Electrical/Electrical Elements/Switch  R_closed=nmqmxcdyxn Ohm  G_open=sifsbhriko 1/Ohm  Threshold=uenjiusouk  i_specify=off  i_priority=None  i=vnemzslczv A  i_nominal_specify=off  i_nominal_unit=A  i_nominal_value=qcfwbklixv  v_specify=off  v_priority=None  v=kbptsqwrrs V  v_nominal_specify=off  v_nominal_unit=V  v_nominal_value=oanrndtlko
      settings: SourceProductName=Simscape
  Redacted_5158 : ee_lib/Passive/Thermal/Thermal Resistor  R=googadkadv K/W  T_specify=off  T_priority=None  T=qvfxxsvwyd K  T_nominal_specify=off  T_nominal_unit=K  T_nominal_value=utalmaxmos  Q_specify=off  Q_priority=None  Q=ozoenihjte W  Q_nominal_specify=off  Q_nominal_unit=W  Q_nominal_value=kxajlgzitx
      settings: SourceProductName=Simscape Electrical  SourceProductBaseCode=PS  InternalSimscapePortConfiguration="{\"Bottom\":[],\"Left\":[{\"id\":\"A\",\"label\":\"A\",\"type\":\"foundation.thermal.thermal\"}],\"Right\":[{\"id\":\"B\",\"label\":\"B\",\"type\":\"foundation.thermal.thermal\"}],\"Top\":[]}"
  Redacted_6192 : ee_lib/Semiconductors & Converters/Diode  ModelType=wjaiuhkfjd  Vf=wgohbbjtou V  Ron=jwlotyysxe Ohm  Goff=fdbijllkro S  prmExp=wygvsfrlui  I12=qkyqevrabk A  V12=rulzmosgfk V  IS=gzgknqicjl A  ec=echudalzbj  I1=iucxputfsn A  V1=urphrudfbq V  RS=vungouopdq Ohm  Tmeas=rfdetovvtm degC  N_series=tfugmmptwz  N_parallel=zmbqbfqnfe  Rz=reibdskuxy Ohm  BV=ehwapyqchw V  C_param=uhefoqkvit  CJ=xnkbufkgwv pF  CJ0=ilfzdqyspz pF  VJ=qacqnepjof V  Mgrad=ogdccqnzcv  Vvec=qkiwicjtyv V  Cvec=tsettqepzz pF  FC=xspzaalgge  Q_param=lxrxczaxsb  iRM=vxculdednk A  iF=bgqnoqcung A  didt=jcghdrslyf A/us  trr_factor=vydqqumurm  trr=clpyydxtuk ns  Qrr=dmvddbskmb s*uA  TT=sdpvwflaoi ns  tau=inilbkpskq ns  T_param=aftqnzwbwk  IS_T2=zhthrzvtbc A  I1_T2=kvowpjkfkh A  V1_T2=utefudyuay V  Tmeas2=rnmkkaylmd degC  EG_param=rxkmndinal  EG=qyqdsuyjju eV  XTI_param=bnzclodezw  XTI=dsvgwllmmr  dBVdT=xvvfmlntlp V/K  Tdevice=teetxpjmjc degC  i_specify=off  i_priority=None  i=ejmyycllhz A  i_nominal_specify=off  i_nominal_unit=A  i_nominal_value=upnsogywoc  v_specify=off  v_priority=None  v=iszehztdti V  v_nominal_specify=off  v_nominal_unit=V  v_nominal_value=xjeiqlehrg  i_capacitor_specify=off  i_capacitor_priority=None  i_capacitor=mabsqroqgg A  i_capacitor_nominal_specify=off  i_capacitor_nominal_unit=A  i_capacitor_nominal_value=eumyxqahsv  v_capacitor_specify=off  v_capacitor_priority=None  v_capacitor=mbbbuvuywc V  v_capacitor_nominal_specify=off  v_capacitor_nominal_unit=V  v_capacitor_nominal_value=vbgelovtxw  power_dissipated_specify=off  power_dissipated_priority=None  power_dissipated=xdloyluync W  power_dissipated_nominal_specify=off  power_dissipated_nominal_unit=W  power_dissipated_nominal_value=zqfulfzrvg  thermal_network_parameterization=eqpajgdrtb  Rth=nlwvhnzaki K/W  Rth_Foster=ceczlandcr K/W  thermal_mass_parameterization=gesjogfdkp  thermal_mass=nwzcqrnrer J/K  thermal_mass_Foster=ystvavtqvz J/K  thermal_time_constant=lcsdrnwpuk s  thermal_time_constant_Foster=cwkrlebhqf s  thermal_mass_initial_temperatures=vqomqkaabf degC
      settings: SourceProductName=Simscape Electrical  InternalSimscapePortConfiguration="{\"Bottom\":[],\"Left\":[{\"id\":\"p\",\"label\":\"\",\"type\":\"foundation.electrical.electrical\"},{\"id\":\"H\",\"label\":\"H\",\"type\":\"foundation.thermal.thermal\"}],\"Right\":[{\"id\":\"n\",\"label\":\"\",\"type\":\"foundation.electrical.electrical\"}],\"Top\":[]}"
  Redacted_8464 : fl_lib/Electrical/Electrical Elements/Switch  R_closed=iphoajggoa Ohm  G_open=cwcrdsoguf 1/Ohm  Threshold=uurnpckbxo  i_specify=off  i_priority=None  i=otavnsrwfy A  i_nominal_specify=off  i_nominal_unit=A  i_nominal_value=alcwmabqzx  v_specify=off  v_priority=None  v=dkrggmbjgc V  v_nominal_specify=off  v_nominal_unit=V  v_nominal_value=agmihkmkxp
      settings: SourceProductName=Simscape
  Redacted_912 : ee_lib/Semiconductors & Converters/Diode  ModelType=iglazncixp  Vf=bkwghmjgog V  Ron=ubscuoanxv Ohm  Goff=spdmgthuhd S  prmExp=vypqjycbuv  I12=nalsffqkra A  V12=mhtzatimml V  IS=ozislkwjvv A  ec=pglttnlnce  I1=kyieltmplt A  V1=eltyboevkb V  RS=apsrrfztac Ohm  Tmeas=vxanoodkay degC  N_series=faxhcpsvcs  N_parallel=xxurtqimfq  Rz=bogkpobwiq Ohm  BV=cljeerzocy V  C_param=iuifemeyxs  CJ=wisvvtzgvj pF  CJ0=ewywlmddbo pF  VJ=ysfsdbidrh V  Mgrad=xkyayjxkdt  Vvec=zqbkcfkkwh V  Cvec=pkenprsxno pF  FC=enqlzcdqjg  Q_param=qhbgcmjkih  iRM=eutdgogkuj A  iF=wribsrpddt A  didt=njzthozsez A/us  trr_factor=sopcwwixbo  trr=bdeciguydj ns  Qrr=icdmoamdts s*uA  TT=nbagowlmyq ns  tau=bdggqoohns ns  T_param=jzdlenyiae  IS_T2=nammcxgudj A  I1_T2=fbqdllpxxu A  V1_T2=olpoomlehh V  Tmeas2=hvtlifamgm degC  EG_param=rwxchefnjv  EG=vfiskjbokw eV  XTI_param=lcxreednpx  XTI=stufcfgqtt  dBVdT=ecziobvzqs V/K  Tdevice=hqhpmhjats degC  i_specify=off  i_priority=None  i=zokpqmswev A  i_nominal_specify=off  i_nominal_unit=A  i_nominal_value=sqhefqjfkm  v_specify=off  v_priority=None  v=kkoieydcvv V  v_nominal_specify=off  v_nominal_unit=V  v_nominal_value=xdzjgytxkz  i_capacitor_specify=off  i_capacitor_priority=None  i_capacitor=mjhdqpjpvl A  i_capacitor_nominal_specify=off  i_capacitor_nominal_unit=A  i_capacitor_nominal_value=olycbrmlpz  v_capacitor_specify=off  v_capacitor_priority=None  v_capacitor=klssxycbgm V  v_capacitor_nominal_specify=off  v_capacitor_nominal_unit=V  v_capacitor_nominal_value=clqocrvrjh  power_dissipated_specify=off  power_dissipated_priority=None  power_dissipated=tazlifuteu W  power_dissipated_nominal_specify=off  power_dissipated_nominal_unit=W  power_dissipated_nominal_value=xwnjddqcij  thermal_network_parameterization=knxqfzohjn  Rth=hohavsbqch K/W  Rth_Foster=qhckcxiiow K/W  thermal_mass_parameterization=mwwycjxwca  thermal_mass=pmatgnmqzt J/K  thermal_mass_Foster=pruwraeayl J/K  thermal_time_constant=vcteuzqhja s  thermal_time_constant_Foster=dzswwdwfdd s  thermal_mass_initial_temperatures=ulpynusrfs degC
      settings: SourceProductName=Simscape Electrical  InternalSimscapePortConfiguration="{\"Bottom\":[],\"Left\":[{\"id\":\"p\",\"label\":\"\",\"type\":\"foundation.electrical.electrical\"},{\"id\":\"H\",\"label\":\"H\",\"type\":\"foundation.thermal.thermal\"}],\"Right\":[{\"id\":\"n\",\"label\":\"\",\"type\":\"foundation.electrical.electrical\"}],\"Top\":[]}"
  Redacted_2150 : PMIOPort  Side=Left
  Redacted_3412 : PMIOPort  Port=2  Side=Right
  Redacted_2301 : PMIOPort  Port=3  Side=Left
  Redacted_7111 : PMIOPort  Port=4  Side=Right
  Redacted_733 : PMIOPort  Port=5  Side=Left
  Redacted_3824 : PMIOPort  Port=6  Side=Right
  connections:
  Redacted_8464/LConn1 -- Redacted_1604/LConn1 -- Redacted_912/RConn1
  Redacted_912/LConn1 -- Redacted_2301/RConn1 -- Redacted_1604/RConn1
  Redacted_3309/RConn1 -- Redacted_5158/RConn1 -- Redacted_1380/LConn1
  Redacted_7111/RConn1 -- Redacted_8464/RConn2
  Redacted_3785/RConn1 -- Redacted_3824/RConn1 -- Redacted_8464/RConn1
  Redacted_3412/RConn1 -- Redacted_3785/RConn2
  Redacted_6192/LConn1 -- Redacted_3785/LConn1 -- Redacted_2923/RConn1
  Redacted_2923/LConn1 -- Redacted_2150/RConn1 -- Redacted_6192/RConn1
  Redacted_5158/LConn1 -- Redacted_1604/LConn2 -- Redacted_912/LConn2
  Redacted_1380/RConn1 -- Redacted_733/RConn1
  Redacted_3309/LConn1 -- Redacted_2923/LConn2 -- Redacted_6192/LConn2
